simulink model "ex5"  (R2022a)
settings: Solver=VariableStepAuto  StartTime=0.0  StopTime=25  RelTol=1e-3
values from neighbouring files (symbols this model uses):
  D = 2 * sqrt((fx+Kp)*Mx)    [ex5mat.m]
  Do = 2 * sqrt((mud+Ko)*Mo)    [ex5mat.m]
  dt = 0.01    [EulerAngleController.m]    (also in ex5mat.m)
  fd = [5 0 0]    [ex5mat.m]
  K = [1 0 0; 0 0.5 0; 0 0 1]    [EulerAngleController.m]    (also in ex5mat.m = [10 0 0; 0 0 0; 0 0 0])
  Kf = [0.075 0 0; 0 1 0; 0 0 1]    [ex5mat.m]
  Ki = [0.01 0 0; 0 1 0; 0 0 1]    [ex5mat.m]
  Ko = [2 0 0; 0 1 0; 0 0 2]    [ex5mat.m]
  Kp = [2 0 0; 0 1 0; 0 0 2]    [ex5mat.m]
  Minv = inv(Mx)    [ex5mat.m]
  Moinv = inv(Mo)    [ex5mat.m]
libraries: robotcorelib x2, aerolibutil x1
settings Model: Creator=marcu  LastModifiedBy=marcu
settings DebuggingCC: UnconnectedInputMsg=warning  UnconnectedOutputMsg=warning  UnconnectedLineMsg=warning
settings RTWCC: DLArmComputeVersion=19.05

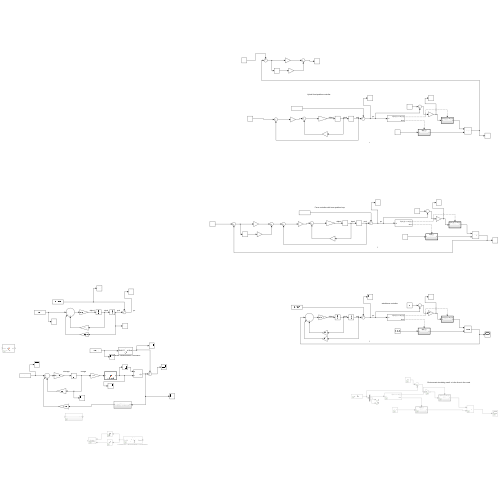
[thumbnail: Simulink's stored preview of the top-level diagram]
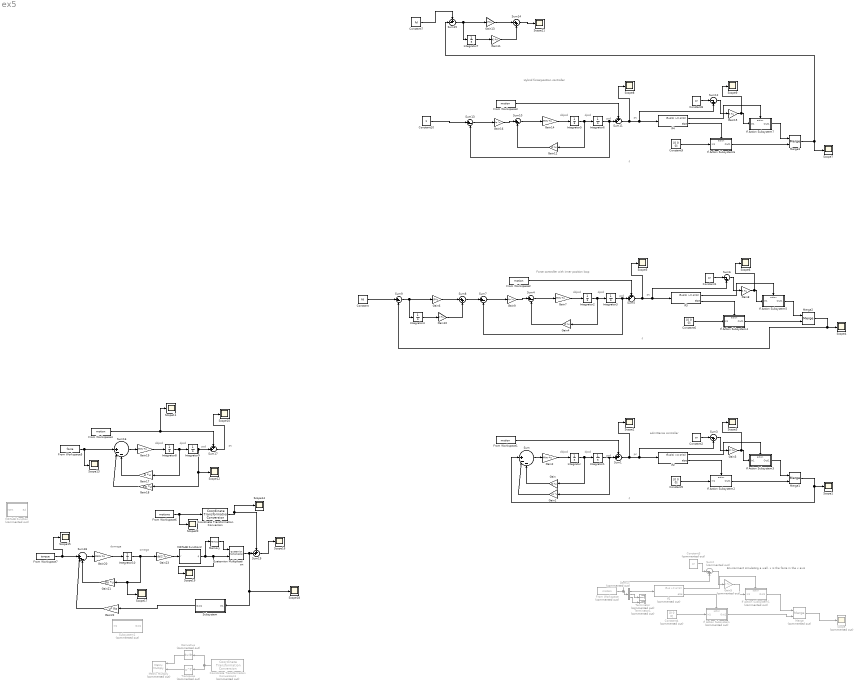
== system ex5 ==
  note: omega
  note: domega
  note: Hybrid force/position controller
  note: Force controller with inner position loop
  note: admittance controller
  note: Environment simulating a wall. x is the force in the x axis
  note: f
  note: pc
  note: pcd
  note: dpcd
  note: ddpcd
  note: f
  note: pcd
  note: dpcd
  note: ddpcd
  note: pc
  note: pc
  note: ddpcd
  note: pcd
  note: dpcd
  note: f
  note: pcd
  note: dpcd
  note: ddpcd
  note: pc
  Constant : Constant  Value=fd
  Constant1 : Constant  Value=or
  Constant10 : Constant
  Constant2 : Constant  Value=or
  Constant3 : Constant  Commented=on  Value=or
  Constant4 : Constant  Commented=on  Value=[0 0 0]
  Constant5 : Constant  Value=[0 0 0]
  Constant6 : Constant  Value=[0 0 0]
  Constant7 : Constant  Value=fd
  Constant8 : Constant  Value=or
  Constant9 : Constant  Value=[0 0 0]
  Coordinate Transformation Conversion : robotcorelib/Coordinate Transformation Conversion  InputRepresentation=Euler Angles  InputEulerSequence=XYZ  ShowTrVecInputPort=on  OutputRepresentation=Quaternion  OutputEulerSequence=ZYX  ShowTrVecOutputPort=on  SimulateUsing=Interpreted execution
      settings: SourceProductBaseCode=RO,NV,RR,UV
  Coordinate Transformation Conversion1 : robotcorelib/Coordinate Transformation Conversion  Commented=on  InputRepresentation=Quaternion  InputEulerSequence=ZYX  ShowTrVecInputPort=on  OutputRepresentation=Rotation Matrix  OutputEulerSequence=ZYX  ShowTrVecOutputPort=on  SimulateUsing=Interpreted execution
      settings: SourceProductBaseCode=RO,NV,RR,UV
  Demux : Demux  Commented=on  Outputs=3
  Derivative : Derivative  Commented=on
  From Workspace : FromWorkspace  Commented=on  VariableName=motion
  From Workspace{1..4} (4 alike) : FromWorkspace  VariableName=motion
  From Workspace5 : FromWorkspace  VariableName=force
  From Workspace6 : FromWorkspace  VariableName=motiono
  From Workspace7 : FromWorkspace  VariableName=torque
  Gain{,4,12,17} (4 alike) : Gain  Gain=D  Multiplication=Matrix(K*u)
  Gain{1,9,16,18} (4 alike) : Gain  Gain=Kp  Multiplication=Matrix(K*u)
  Gain10 : Gain  Gain=Ki  Multiplication=Matrix(K*u)
  Gain11 : Gain  Gain=Ki  Multiplication=Matrix(K*u)
  Gain13 : Gain  Gain=Kf  Multiplication=Matrix(K*u)
  Gain{2,7,14,19} (4 alike) : Gain  Gain=Minv  Multiplication=Matrix(K*u)
  Gain15 : Gain  Gain=K  Multiplication=Matrix(K*u)
  Gain20 : Gain  Gain=Moinv  Multiplication=Matrix(K*u)
  Gain21 : Gain  Gain=Do  Multiplication=Matrix(K*u)
  Gain22 : Gain  Gain=Ko  Multiplication=Matrix(u*K)
  Gain23 : Gain  Gain=dt/2  Multiplication=Matrix(K*u)
  Gain3 : Gain  Gain=-K  Multiplication=Matrix(K*u)
  Gain5 : Gain  Commented=on  Gain=K  Multiplication=Matrix(K*u)
  Gain6 : Gain  Gain=Kf  Multiplication=Matrix(K*u)
  Gain8 : Gain  Gain=K  Multiplication=Matrix(K*u)
  If Action Subsystem : Subsystem  Commented=on  TreatAsAtomicUnit=on
  If Action Subsystem1 : Subsystem  Commented=on  TreatAsAtomicUnit=on
  If Action Subsystem2 : Subsystem  TreatAsAtomicUnit=on
  If Action Subsystem3 : Subsystem  TreatAsAtomicUnit=on
  If Action Subsystem4 : Subsystem  TreatAsAtomicUnit=on
  If Action Subsystem5 : Subsystem  TreatAsAtomicUnit=on
  If Action Subsystem6 : Subsystem  TreatAsAtomicUnit=on
  If Action Subsystem7 : Subsystem  TreatAsAtomicUnit=on
  If1 : If  Commented=on  IfExpression=u1 >= or(1)
  If2 : If  IfExpression=u1(1) >= or(1)
  If3 : If  IfExpression=u1(1) >= or(1)
  If4 : If  IfExpression=u1(1) >= or(1)
  Integrator{,1..10} (11 alike) : Integrator
  MATLAB Function : MATLAB Function  Commented=on  TreatAsAtomicUnit=on
  MATLAB Function2 : MATLAB Function  TreatAsAtomicUnit=on
  Matrix Multiply : Product  Commented=on  Multiplication=Matrix(*)
  Memory : Memory
  Merge : Merge  Commented=on
  Merge1 : Merge
  Merge2 : Merge
  Merge3 : Merge
  Quaternion Multiplication : aerolibutil/Quaternion Multiplication
  Scope : Scope  Commented=on
  Scope{1..21} (21 alike) : Scope
  Subsystem : Subsystem
  Subsystem1 : Subsystem  Commented=on
  Sum : Sum  Inputs=||+--
  Sum{1,5,11,17,19} (5 alike) : Sum  Inputs=++|
  Sum{4,7,9..10,13} (5 alike) : Sum  Inputs=|+-
  Sum12 : Sum  Inputs=|-+
  Sum14 : Sum  Inputs=|++
  Sum15 : Sum  Inputs=+-|
  Sum16 : Sum  Inputs=||+--
  Sum18 : Sum  Inputs=||+--
  Sum2 : Sum  Commented=on  Inputs=|-+
  Sum3 : Sum  Inputs=|-+
  Sum6 : Sum  Inputs=|-+
  Sum8 : Sum  Inputs=|++
  Terminator : Terminator  Commented=on
  Terminator1 : Terminator  Commented=on
  Transpose : Math  Commented=on  Operator=transpose
  wires:
  Gain/1 -> Sum/3
  Gain1/1 -> Sum/2
  Sum/1 -> Gain2/1
  Gain2/1 -> Integrator/1
  Integrator/1 -> Gain/1, Integrator1/1
  Integrator1/1 -> Gain1/1, Sum1/2
  From Workspace1/1 -> Sum1/1
  From Workspace/1 -> Sum2/2, Demux/1
  If1/2 -> If Action Subsystem/Action
  If1/1 -> If Action Subsystem1/Action
  Constant3/1 -> Sum2/1
  Sum2/1 -> Gain5/1
  Demux/1 -> If1/1
  Demux/2 -> Terminator/1
  Demux/3 -> Terminator1/1
  If Action Subsystem/1(Out1) -> Merge/2
  Constant4/1 -> If Action Subsystem/1(In1)
  Gain5/1 -> If Action Subsystem1/1(In1)
  If Action Subsystem1/1(Out1) -> Merge/1
  Merge/1 -> Scope/1
  Constant5/1 -> If Action Subsystem2/1(In1)
  If Action Subsystem3/1(Out1) -> Merge1/1
  Gain3/1 -> Scope3/1, If Action Subsystem3/1(In1)
  If Action Subsystem2/1(Out1) -> Merge1/2
  Sum1/1 -> Scope2/1, If2/1, Sum3/2
  If2/1 -> If Action Subsystem3/Action
  Constant2/1 -> Sum3/1
  Sum3/1 -> Gain3/1
  If2/2 -> If Action Subsystem2/Action
  Merge1/1 -> Sum/1, Scope1/1
  From Workspace2/1 -> Sum5/1
  Constant6/1 -> If Action Subsystem4/1(In1)
  Sum5/1 -> Scope5/1, If3/1, Sum6/2
  If3/2 -> If Action Subsystem4/Action
  If3/1 -> If Action Subsystem5/Action
  Constant1/1 -> Sum6/1
  Sum6/1 -> Gain8/1
  Merge2/1 -> Sum9/2, Scope4/1
  Sum4/1 -> Gain7/1
  If Action Subsystem5/1(Out1) -> Merge2/1
  Gain8/1 -> Scope6/1, If Action Subsystem5/1(In1)
  Integrator3/1 -> Sum7/2, Sum5/2
  Integrator2/1 -> Gain4/1, Integrator3/1
  Gain7/1 -> Integrator2/1
  Gain4/1 -> Sum4/2
  If Action Subsystem4/1(Out1) -> Merge2/2
  Gain9/1 -> Sum4/1
  Sum7/1 -> Gain9/1
  Sum8/1 -> Sum7/1
  Gain6/1 -> Sum8/1
  Gain10/1 -> Sum8/2
  Integrator4/1 -> Gain10/1
  Sum9/1 -> Integrator4/1, Gain6/1
  Constant/1 -> Sum9/1
  Constant7/1 -> Sum15/1
  Gain16/1 -> Sum10/1
  Gain12/1 -> Sum10/2
  Sum10/1 -> Gain14/1
  Sum15/1 -> Integrator7/1, Gain13/1
  If Action Subsystem6/1(Out1) -> Merge3/2
  Sum13/1 -> Gain16/1
  Gain14/1 -> Integrator5/1
  Merge3/1 -> Scope7/1, Sum15/2
  Gain15/1 -> Scope9/1, If Action Subsystem7/1(In1)
  If Action Subsystem7/1(Out1) -> Merge3/1
  Integrator6/1 -> Sum13/2, Sum11/2
  If4/1 -> If Action Subsystem7/Action
  Sum12/1 -> Gain15/1
  If4/2 -> If Action Subsystem6/Action
  Constant8/1 -> Sum12/1
  Integrator5/1 -> Gain12/1, Integrator6/1
  Sum11/1 -> Scope8/1, If4/1, Sum12/2
  From Workspace3/1 -> Sum11/1
  Gain11/1 -> Sum14/2
  Constant9/1 -> If Action Subsystem6/1(In1)
  Gain13/1 -> Sum14/1
  Integrator7/1 -> Gain11/1
  From Workspace4/1 -> Scope11/1, Sum17/1
  Sum17/1 -> Scope10/1
  Gain17/1 -> Sum16/3
  Gain19/1 -> Integrator8/1
  Sum16/1 -> Gain19/1
  Gain18/1 -> Sum16/2
  Integrator8/1 -> Gain17/1, Integrator9/1
  From Workspace5/1 -> Sum16/1, Scope13/1
  Integrator9/1 -> Sum17/2, Scope12/1, Gain18/1
  From Workspace7/1 -> Scope15/1, Sum18/1
  From Workspace6/1 -> Coordinate Transformation Conversion/1, Scope20/1
  Sum19/1 -> Scope16/1
  Sum18/1 -> Gain20/1
  Gain20/1 -> Integrator10/1
  Gain21/1 -> Sum18/3
  Gain22/1 -> Sum18/2
  Integrator10/1 -> Gain23/1, Scope17/1, Gain21/1
  Gain23/1 -> MATLAB Function2/1(r)
  MATLAB Function2/1(q) -> Quaternion Multiplication/2, Scope19/1, Memory/1
  Quaternion Multiplication/1 -> Subsystem/1(In1), Scope18/1, Sum19/2
  Memory/1 -> Quaternion Multiplication/1
  Coordinate Transformation Conversion/1 -> Sum19/1, Scope14/1
  Coordinate Transformation Conversion1/1 -> Transpose/1, Derivative/1
  Derivative/1 -> Matrix Multiply/1
  Transpose/1 -> Matrix Multiply/2
  Subsystem/1(Out1) -> Gain22/1
  Constant10/1 -> Sum13/1
  Sum14/1 -> Scope21/1

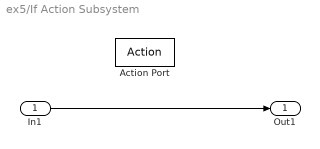
== system ex5/If Action Subsystem ==
  In1 : Inport
  Action Port : ActionPort  ActionPortLabel=else
  Out1 : Outport
  wires:
  In1/1 -> Out1/1

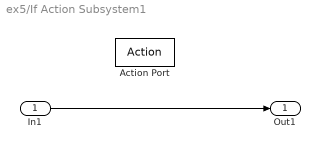
== system ex5/If Action Subsystem1 ==
  In1 : Inport
  Action Port : ActionPort  ActionPortLabel=if(u1 >= or(1))
  Out1 : Outport
  wires:
  In1/1 -> Out1/1

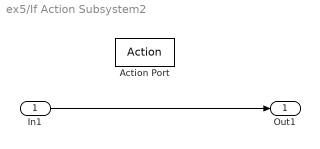
== system ex5/If Action Subsystem2 ==
  In1 : Inport
  Action Port : ActionPort  ActionPortLabel=else
  Out1 : Outport
  wires:
  In1/1 -> Out1/1

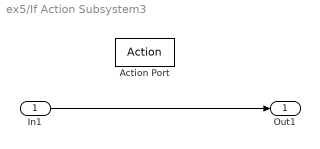
== system ex5/If Action Subsystem3 ==
  In1 : Inport
  Action Port : ActionPort  ActionPortLabel=if(u1(1) >= or(1))
  Out1 : Outport
  wires:
  In1/1 -> Out1/1

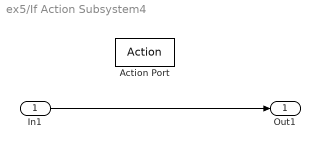
== system ex5/If Action Subsystem4 ==
  In1 : Inport
  Action Port : ActionPort  ActionPortLabel=else
  Out1 : Outport
  wires:
  In1/1 -> Out1/1

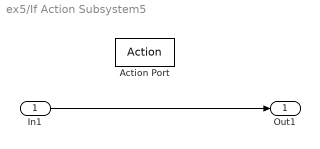
== system ex5/If Action Subsystem5 ==
  In1 : Inport
  Action Port : ActionPort  ActionPortLabel=if(u1(1) >= or(1))
  Out1 : Outport
  wires:
  In1/1 -> Out1/1

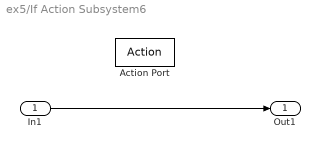
== system ex5/If Action Subsystem6 ==
  In1 : Inport
  Action Port : ActionPort  ActionPortLabel=else
  Out1 : Outport
  wires:
  In1/1 -> Out1/1

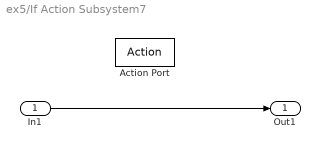
== system ex5/If Action Subsystem7 ==
  In1 : Inport
  Action Port : ActionPort  ActionPortLabel=if(u1(1) >= or(1))
  Out1 : Outport
  wires:
  In1/1 -> Out1/1

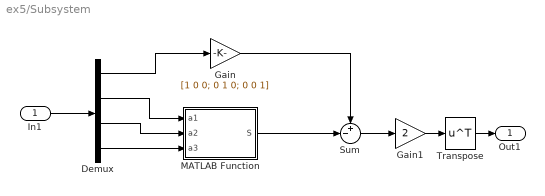
== system ex5/Subsystem ==
  In1 : Inport
  Demux : Demux
  Gain : Gain  Gain=[1 0 0; 0 1 0; 0 0 1]
  Gain1 : Gain  Gain=2
  MATLAB Function : MATLAB Function  TreatAsAtomicUnit=on
  Sum : Sum  Inputs=+-|
  Transpose : Math  Operator=transpose
  Out1 : Outport
  wires:
  In1/1 -> Demux/1
  Gain/1 -> Sum/1
  Demux/1 -> Gain/1
  Demux/2 -> MATLAB Function/1(a1)
  Demux/3 -> MATLAB Function/2(a2)
  Demux/4 -> MATLAB Function/3(a3)
  MATLAB Function/1(S) -> Sum/2
  Sum/1 -> Gain1/1
  Gain1/1 -> Transpose/1
  Transpose/1 -> Out1/1

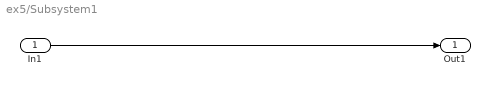
== system ex5/Subsystem1 ==
  In1 : Inport
  Out1 : Outport
  wires:
  In1/1 -> Out1/1

== matlab function ex5/MATLAB Function ==
  data: rotm input; eul output
function eul = rot2eul(rotm)
rotmeul = [0 -rotm(3) rotm(2); rotm(3) 0 -rotm(1); -rotm(2) rotm(1) 0];
eul = rotm2eul(rotmeul);

== matlab function ex5/MATLAB Function2 ==
  data: r input; q output
function q = vel2quat(r)

n = cos(norm(r));
e = (r/norm(r)).*sin(r);

q = [n e']';

== matlab function ex5/Subsystem/MATLAB Function ==
  data: a1 input; S output; a2 input; a3 input
function S = fcn(a1, a2, a3)

S = [0 -a3 a2; a3 0 -a1; -a2 a1 0];
